simulink model "Controller_implementation"  (R2024a)
settings: Solver=FixedStepAuto  StartTime=0.0  StopTime=inf  RelTol=1e-3  EnableMultiTasking=on
values from neighbouring files (symbols this model uses):
  dis = 81.17 * 10^-3    (= 0.08117)    [Motormixing.m]
  drag_co = torque_Nm / no_rot^2    (= 9.75332775919e-12)    [QuadcopterAttributes.m]
  F = [1 0 0 0 0 0 0 0 ... (first row only)    [LQI_reduced.m]
  g = 9.81    [StateSpace.m]
  K_D_LQR_reduced = lqrd(A_r, B_r, Q_reduced, R_reduced, Ts)    [discrete_control.m]
  K_mm = inv(K_mm_FtoU)    [Motormixing.m]
  Ki_D_lqi_reduced_a = K_lqi_reduced_a(:,9:12)    [discrete_control.m]
  KV_rating = 2800    [QuadcopterAttributes.m]
  Kx_D_lqi_reduced_a = K_lqi_reduced_a(:,1:8)    [discrete_control.m]
  lift_co = thrust_N / no_rot^2    (= 5.88883004597e-10)    [QuadcopterAttributes.m]
  m = 0.5    [StateSpace.m]
  R_kalman = diag([variance_Height, variance_rollAngle, variance_pitchAngle, variance_Yaw, variance_GyroRoll, variance_GyroPitch, variance_GyroYaw])    [BBB_calibration_dev2.m]    (also in Kalman.m = [1 0 0 0 0 0 0)
  Ts = 0.01    [discrete_control.m]
undefined symbols (not defined in the file or in its folder): A_r_d, B_r_d, battery_voltage, C_r_d, D_r_d, DiscIntNeverNeededParam, Discrete, Time
libraries: bbblueActuatorLib x4, simulink_extras x2, bbblueSensorLib x2, ctrlSharedLib x1, dspstat3 x1, dspsigops x1
settings Model: SimulationMode=external  ExtModeTrigDuration=100  Creator=Dario  LastModifiedBy=Henrik
settings SolverCC: PositivePriorityOrder=on
settings OptimizationCC: EnhancedBackFolding=on  PassReuseOutputArgsAs=Individual arguments  ZeroExternalMemoryAtStartup=off  ZeroInternalMemoryAtStartup=off  MaxStackSize=64  OptimizeBlockOrder=speed  DifferentSizesBufferReuse=on  OptimizationCustomize=off  EfficientTunableParamExpr=on
settings DebuggingCC: ParameterTunabilityLossMsg=error
settings HardwareCC: ProdBitPerPointer=32  ProdBitPerSizeT=32  ProdBitPerPtrDiffT=32  ProdLargestAtomicInteger=Long  ProdLargestAtomicFloat=Double  ProdWordSize=32  ProdHWDeviceType=ARM Compatible->ARM Cortex
settings SFSimCC: MATLABDynamicMemAlloc=off
settings RTWCC: Description=Embedded Coder  SystemTargetFile=ert.tlc  HardwareBoard=BeagleBone Blue  TLCOptions="-aInlineSetEventsForThisBaseRateFcn=TLC_FALSE -aSuppressMultiTaskScheduler=TLC_FALSE  -aRateBasedStepFcn=0"  TemplateMakefile=ert_default_tmf  Toolchain=GNU GCC BeagleBone Blue
settings CodeAppCC: ForceParamTrailComments=on  IgnoreCustomStorageClasses=off  OperatorAnnotations=on  SimulinkDataObjDesc=on  SFDataObjDesc=on  InsertBlockDesc=on
settings ERTTargetCC: SupportVariableSizeSignals=on  ExtMode=on  ExtModeMexArgs='192.168.7.2' 0 17725

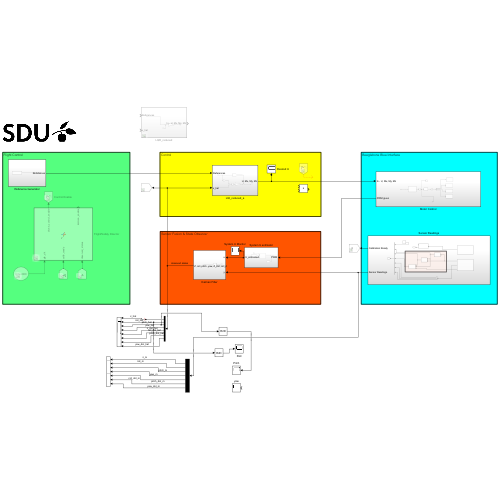
[thumbnail: Simulink's stored preview of the top-level diagram]
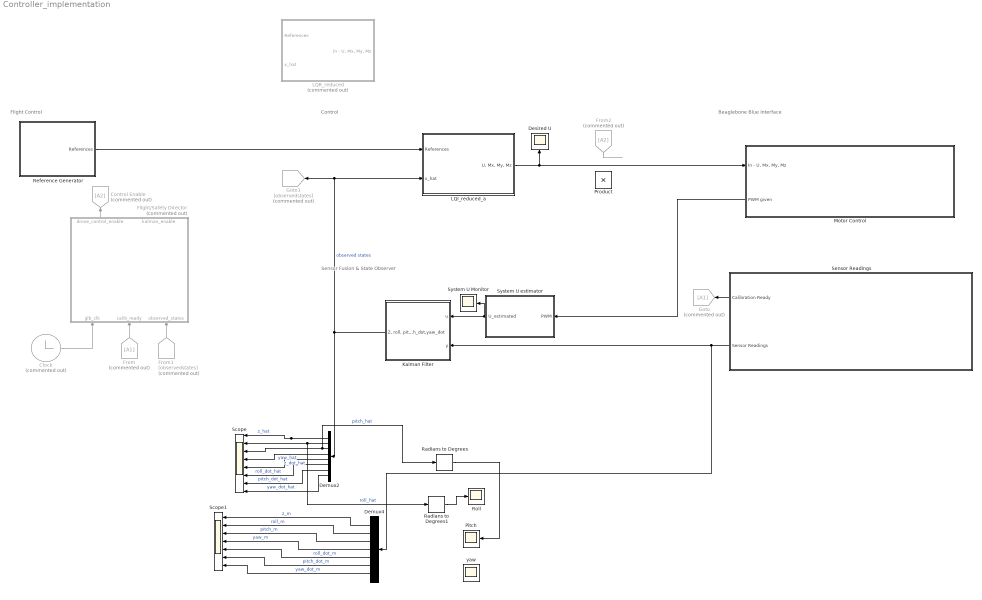
== system Controller_implementation ==
  note: Flight Control
  note: Sensor Fusion & State Observer
  note: Control
  note: Beaglebone Blue Interface
  Clock : Clock  Commented=on
  Control Enable : Goto  Commented=on  GotoTag=A2
  Demux2 : Demux  Outputs=8
  Demux4 : Demux  Outputs=7
  Desired U : Scope
  Flight/Safety Director : MATLAB Function  Commented=on  TreatAsAtomicUnit=on
  From : From  Commented=on  GotoTag=A1
  From1 : From  Commented=on  GotoTag=observedstates
  From2 : From  Commented=on  GotoTag=A2
  Goto : Goto  Commented=on  GotoTag=A1
  Goto1 : Goto  Commented=on  GotoTag=observedstates
  Kalman Filter : Subsystem
  LQI_reduced_a : Subsystem
  LQR_reduced : Subsystem  Commented=on
  Motor Control : Subsystem
      settings: PortSchema="{\"entries\":[{\"content\":{\"sides\":[{\"content\":{\"connectorIds\":[\"In1\",\"Out1\"]},\"type\":\"ConnectorPlacement.EquallySpacedRectSide\",\"uuid\":\"9438d2e9-c32b-4318-b34d-015e09a6ab33\"},{\"content\":{\"side\":\"RIGHT\"},\"type\":\"ConnectorPlacement.EquallySpacedRectSide\",\"uuid\":\"1f1fa985-23a0-47e9-b845-1a4f67fdad51\"},{\"content\":{\"side\":\"TOP\"},\"type\":\"ConnectorPlacement.EquallySpacedRectSide\",\"uuid\":\"e1dcaf73-051b-42d6-8874-ac3417e8774f\"}]},\"type\":\"ConnectorPlacement.EquallySpacedConnector\",\"uuid\":\"43fb11dd-8e84-4752-aa9e-fc065f28cb2c\"}],\"packageUris\":[\"http://schema.mathworks.com/mf0/Connector/R2020b\"],\"version\":\"1.0\"}"
  Pitch : Scope
  Product : Product
  Radians to Degrees : simulink_extras/Transformations/Radians to Degrees
  Radians to Degrees1 : simulink_extras/Transformations/Radians to Degrees
  Reference Generator : Subsystem
  Roll : Scope
  Scope : Scope  NumInputPorts=8
  Scope1 : Scope  NumInputPorts=7
  Sensor Readings : Subsystem
  System U Monitor : Scope
  System U estimator : Subsystem
  yaw : Scope
  wires:
  Reference Generator/1(References) -> LQI_reduced_a/1(References)
  Demux2/1 -> Scope/1  "z_hat"
  Demux2/2 -> Radians to Degrees1/1, Scope/2  "roll_hat"
  Demux2/3 -> Radians to Degrees/1, Scope/3  "pitch_hat"
  Demux2/4 -> Scope/4  "yaw_hat"
  Demux2/5 -> Scope/5  "z_dot_hat"
  Demux2/6 -> Scope/6  "roll_dot_hat"
  Demux2/7 -> Scope/7  "pitch_dot_hat"
  Demux2/8 -> Scope/8  "yaw_dot_hat"
  System U estimator/1(U_estimated) -> Kalman Filter/1(u), System U Monitor/1
  Demux4/3 -> Scope1/3  "pitch_m"
  Demux4/5 -> Scope1/5  "roll_dot_m"
  Demux4/7 -> Scope1/7  "yaw_dot_m"
  Demux4/6 -> Scope1/6  "pitch_dot_m"
  Demux4/2 -> Scope1/2  "roll_m"
  Demux4/1 -> Scope1/1  "z_m"
  Demux4/4 -> Scope1/4  "yaw_m"
  Radians to Degrees/1 -> Pitch/1
  Radians to Degrees1/1 -> Roll/1
  Sensor Readings/2(Sensor Readings) -> Demux4/1, Kalman Filter/2(y)
  Motor Control/1(PWM given) -> System U estimator/1(PWM)
  Kalman Filter/1("Z, roll, pitch, yaw, Z_dot, roll_dot, pitch_dot,yaw_dot") -> Demux2/1, LQI_reduced_a/2(x_hat), Goto1/1  "observed states"
  Sensor Readings/1(Calibration Ready) -> Goto/1
  From/1 -> Flight/Safety Director/2(calib_ready)
  From1/1 -> Flight/Safety Director/3(observed_states)
  LQI_reduced_a/1("U, Mx, My, Mz") -> Desired U/1, Motor Control/1("In - U, Mx, My, Mz")
  Flight/Safety Director/1(drone_control_enable) -> Control Enable/1
  From2/1 -> ?
  Clock/1 -> Flight/Safety Director/1(glb_clk)

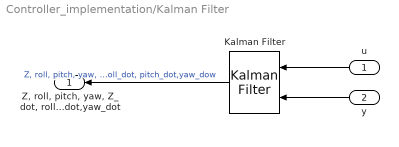
== system Controller_implementation/Kalman Filter ==
  u : Inport
  y : Inport  Port=2
  Kalman Filter : ctrlSharedLib/Kalman Filter  TimeDomain=Discrete-Time  UseCurrentEstimator=on  ModelSource=Individual A, B, C, D matrices  ModelSourceVariable=ss(0.95,1,1,0,1)  A=A_r_d  B=B_r_d  C=C_r_d  D=D_r_d  NumberOfStates=1  NumberOfInputs=1  NumberOfOutputs=1  InitialEstimateSource=Dialog  X0=0  P0=10  UseK=off  UseGH=off  NumberOfProcessNoiseInputs=1  G=1  TimeInvariantG=on  H=0  TimeInvariantH=on  Q=Q_kalman_d  TimeInvariantQ=on  R=R_kalman  TimeInvariantR=on  N=0  TimeInvariantN=on  AddInputPort=on  AddEnablePort=off  OutputEstimatedY=off  OutputP=off  Ts=Ts
  "Z, roll, pitch, yaw, Z_dot, roll_dot, pitch_dot,yaw_dot" : Outport
  wires:
  y/1 -> Kalman Filter/2
  u/1 -> Kalman Filter/1
  Kalman Filter/1 -> "Z, roll, pitch, yaw, Z_dot, roll_dot, pitch_dot,yaw_dot"/1  "Z, roll, pitch, yaw, Z_dot, roll_dot, pitch_dot,yaw_dow"

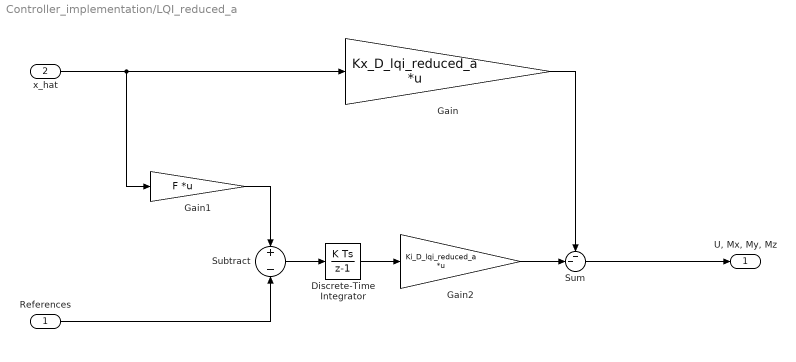
== system Controller_implementation/LQI_reduced_a ==
  References : Inport
  x_hat : Inport  Port=2
  Discrete-Time Integrator : DiscreteIntegrator  SampleTime=Ts  ICPrevOutput=DiscIntNeverNeededParam  ICPrevScaledInput=DiscIntNeverNeededParam
  Gain : Gain  Gain=Kx_D_lqi_reduced_a  Multiplication=Matrix(K*u)
  Gain1 : Gain  Gain=F  Multiplication=Matrix(K*u)
  Gain2 : Gain  Gain=Ki_D_lqi_reduced_a  Multiplication=Matrix(K*u)
  Subtract : Sum  Inputs=+-
  Sum : Sum  Inputs=--|
  "U, Mx, My, Mz" : Outport
  wires:
  Subtract/1 -> Discrete-Time Integrator/1
  Gain1/1 -> Subtract/1
  Sum/1 -> "U, Mx, My, Mz"/1
  Gain/1 -> Sum/1
  Gain2/1 -> Sum/2
  Discrete-Time Integrator/1 -> Gain2/1
  References/1 -> Subtract/2
  x_hat/1 -> Gain/1, Gain1/1

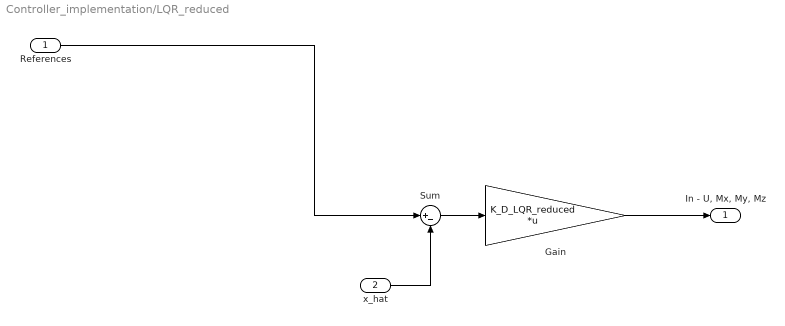
== system Controller_implementation/LQR_reduced ==
  References : Inport
  x_hat : Inport  Port=2
  Gain : Gain  Gain=K_D_LQR_reduced  Multiplication=Matrix(K*u)
  Sum : Sum  Inputs=|+-
  "In - U, Mx, My, Mz" : Outport
  wires:
  Gain/1 -> "In - U, Mx, My, Mz"/1
  Sum/1 -> Gain/1
  References/1 -> Sum/1
  x_hat/1 -> Sum/2

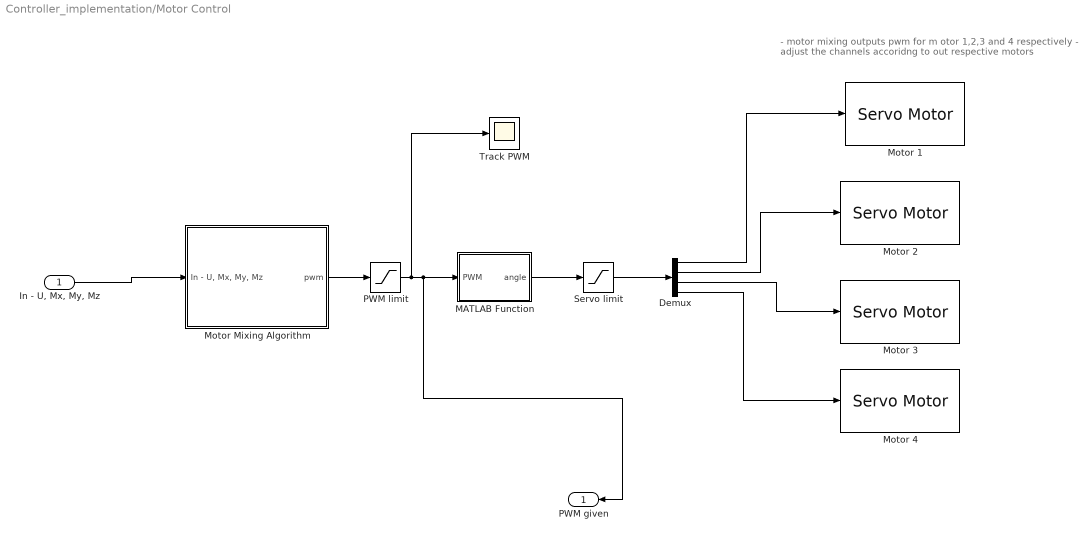
== system Controller_implementation/Motor Control ==
  note: - motor mixing outputs pwm for m otor 1,2,3 and 4 respectively
      | - adjust the channels accoridng to out respective motors
  "In - U, Mx, My, Mz" : Inport
  Demux : Demux
  MATLAB Function : MATLAB Function  TreatAsAtomicUnit=on
  Motor 1 : bbblueActuatorLib/Servo Motor  channel=1  SimulateUsing=Code generation
  Motor 2 : bbblueActuatorLib/Servo Motor  channel=2  SimulateUsing=Code generation
  Motor 3 : bbblueActuatorLib/Servo Motor  channel=3  SimulateUsing=Code generation
  Motor 4 : bbblueActuatorLib/Servo Motor  channel=4  SimulateUsing=Code generation
  Motor Mixing Algorithm : Subsystem
  PWM limit : Saturate  UpperLimit=255  LowerLimit=0
  Servo limit : Saturate  UpperLimit=180  LowerLimit=0
  Track PWM : Scope
  PWM given : Outport
  wires:
  Servo limit/1 -> Demux/1
  PWM limit/1 -> Track PWM/1, PWM given/1, MATLAB Function/1(PWM)
  Demux/4 -> Motor 4/1
  Demux/1 -> Motor 1/1
  Demux/2 -> Motor 2/1
  Motor Mixing Algorithm/1(pwm) -> PWM limit/1
  Demux/3 -> Motor 3/1
  MATLAB Function/1(angle) -> Servo limit/1
  "In - U, Mx, My, Mz"/1 -> Motor Mixing Algorithm/1("In - U, Mx, My, Mz")

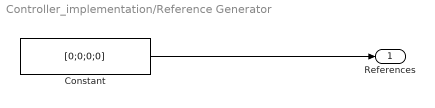
== system Controller_implementation/Reference Generator ==
  Constant : Constant  Value=[0;0;0;0]
  References : Outport
  wires:
  Constant/1 -> References/1

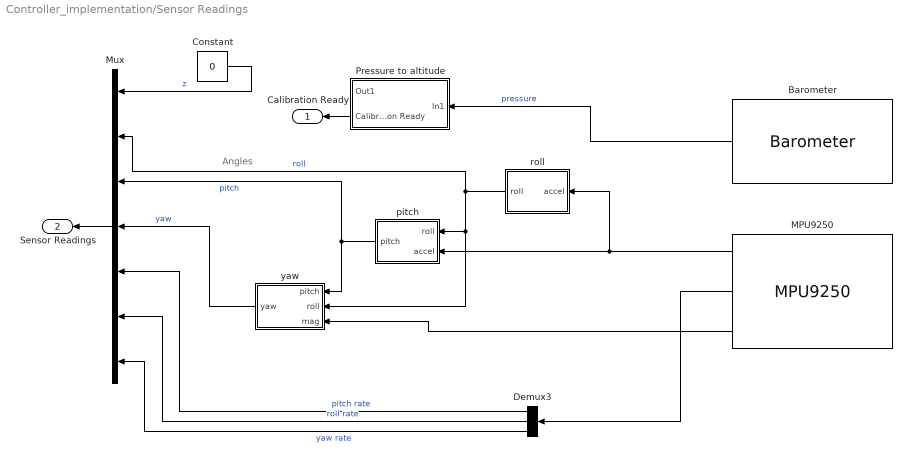
== system Controller_implementation/Sensor Readings ==
  note: Angles
  Barometer : bbblueSensorLib/Barometer  OSRSelection=1  IIRFilterCoeff=Off  SampleTime=Ts
  Constant : Constant  Value=0
  Demux3 : Demux  Outputs=3
  MPU9250 : bbblueSensorLib/MPU9250  OperationMode=DMP  Accel=on  AngularRate=on  Ak8963Field=on  EulerAngles=off  Quat=off  AccelRange=2G  Acceldlpf=1  GyroRange=250 dps  Gyrodlpf=1  DmpOdr=200 Hz  SampleTime=Ts
  Mux : Mux  Inputs=7
  Pressure to altitude : Subsystem
  pitch : MATLAB Function  TreatAsAtomicUnit=on
  "roll " : MATLAB Function  TreatAsAtomicUnit=on
  yaw : MATLAB Function  TreatAsAtomicUnit=on
  Calibration Ready : Outport
  Sensor Readings : Outport  Port=2
  wires:
  Demux3/3 -> Mux/7  "yaw rate"
  yaw/1(yaw) -> Mux/4  "yaw"
  Constant/1 -> Mux/1  "z"
  MPU9250/3 -> yaw/3(mag)
  MPU9250/2 -> Demux3/1
  Demux3/2 -> Mux/6  "roll rate"
  Demux3/1 -> Mux/5  "pitch rate"
  "roll "/1(roll) -> yaw/2(roll), pitch/1(roll), Mux/2  "roll"
  Barometer/1 -> Pressure to altitude/1(In1)  "pressure"
  pitch/1(pitch) -> yaw/1(pitch), Mux/3  "pitch"
  Mux/1 -> Sensor Readings/1
  Pressure to altitude/2(Calibration Ready) -> Calibration Ready/1
  MPU9250/1 -> "roll "/1(accel), pitch/2(accel)

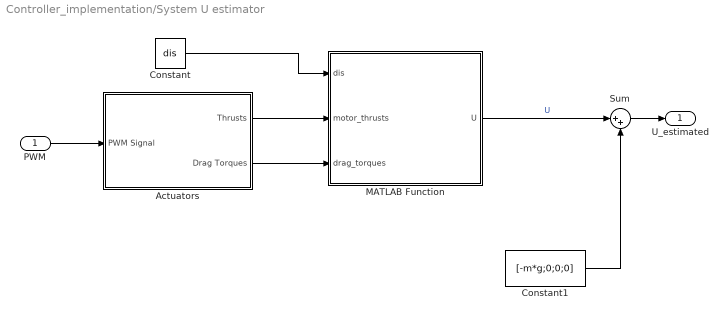
== system Controller_implementation/System U estimator ==
  PWM : Inport
  Actuators : Subsystem
  Constant : Constant  Value=dis
  Constant1 : Constant  Value=[-m*g;0;0;0]  SampleTime=Ts
  MATLAB Function : MATLAB Function  TreatAsAtomicUnit=on
  Sum : Sum  Inputs=|++
  U_estimated : Outport
  wires:
  PWM/1 -> Actuators/1(PWM Signal)
  Actuators/1(Thrusts) -> MATLAB Function/2(motor_thrusts)
  Constant/1 -> MATLAB Function/1(dis)
  Actuators/2(Drag Torques) -> MATLAB Function/3(drag_torques)
  MATLAB Function/1(U) -> Sum/1  "U"
  Constant1/1 -> Sum/2
  Sum/1 -> U_estimated/1

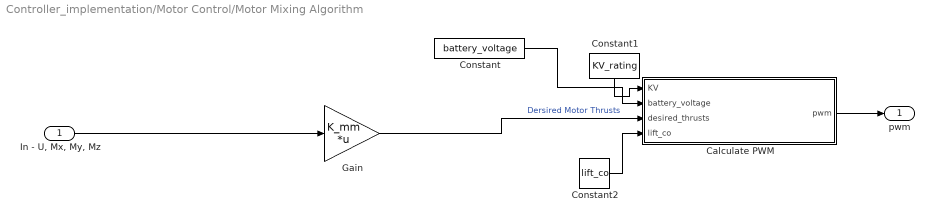
== system Controller_implementation/Motor Control/Motor Mixing Algorithm ==
  "In - U, Mx, My, Mz" : Inport
  Calculate PWM : MATLAB Function  TreatAsAtomicUnit=on
  Constant : Constant  Value=battery_voltage
  Constant1 : Constant  Value=KV_rating
  Constant2 : Constant  Value=lift_co
  Gain : Gain  Gain=K_mm  Multiplication=Matrix(K*u)
  pwm : Outport
  wires:
  "In - U, Mx, My, Mz"/1 -> Gain/1
  Gain/1 -> Calculate PWM/3(desired_thrusts)  "Dersired Motor Thrusts"
  Constant/1 -> Calculate PWM/2(battery_voltage)
  Constant1/1 -> Calculate PWM/1(KV)
  Calculate PWM/1(pwm) -> pwm/1
  Constant2/1 -> Calculate PWM/4(lift_co)

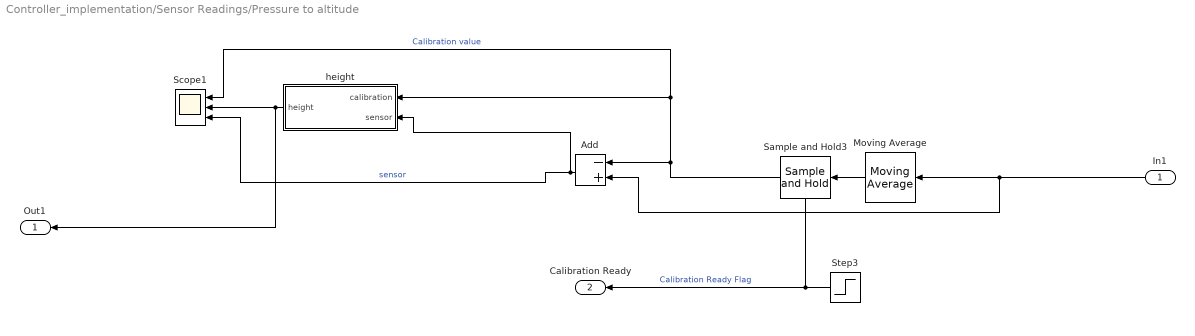
== system Controller_implementation/Sensor Readings/Pressure to altitude ==
  In1 : Inport
  Add : Sum  Inputs=-+
  Moving Average : dspstat3/Moving Average  Method=Exponential weighting  ForgettingFactorPort=off  SpecifyWindowLength=on  WindowLength=4  OverlapLength=3  AllowArbitraryInputLength=off  ForgettingFactor=1.0  SimulateUsing=Code generation
  Sample and Hold3 : dspsigops/Sample and Hold  trig=Rising edge  initCond=100000000  latchinput=off
  Scope1 : Scope  NumInputPorts=3
  Step3 : Step  Time=5  SampleTime=Ts
  height : MATLAB Function  TreatAsAtomicUnit=on
  Out1 : Outport
  Calibration Ready : Outport  Port=2
  wires:
  height/1(height) -> Out1/1, Scope1/2
  Moving Average/1 -> Sample and Hold3/1
  Sample and Hold3/1 -> Scope1/1, height/1(calibration), Add/1  "Calibration value"
  In1/1 -> Add/2, Moving Average/1
  Step3/1 -> Calibration Ready/1, Sample and Hold3/Trigger  "Calibration Ready Flag"
  Add/1 -> height/2(sensor), Scope1/3  "sensor"

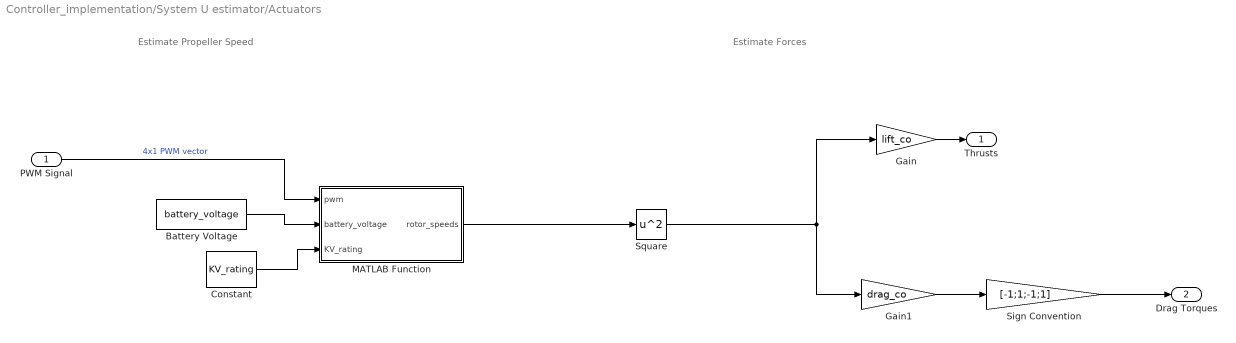
== system Controller_implementation/System U estimator/Actuators ==
  note: Estimate Forces
  note: Estimate Propeller Speed
  PWM Signal : Inport
  Battery Voltage : Constant  Value=battery_voltage  SampleTime=Ts
  Constant : Constant  Value=KV_rating  SampleTime=Ts
  Gain : Gain  Gain=lift_co
  Gain1 : Gain  Gain=drag_co
  MATLAB Function : MATLAB Function  TreatAsAtomicUnit=on
  Sign Convention : Gain  Gain=[-1;1;-1;1]
  Square : Math  Operator=square
  Thrusts : Outport
  Drag Torques : Outport  Port=2
  wires:
  Constant/1 -> MATLAB Function/3(KV_rating)
  Battery Voltage/1 -> MATLAB Function/2(battery_voltage)
  PWM Signal/1 -> MATLAB Function/1(pwm)  "4x1 PWM vector"
  MATLAB Function/1(rotor_speeds) -> Square/1
  Gain/1 -> Thrusts/1
  Square/1 -> Gain/1, Gain1/1
  Gain1/1 -> Sign Convention/1
  Sign Convention/1 -> Drag Torques/1

== matlab function Controller_implementation/System U estimator/Actuators/MATLAB Function ==
  data: pwm input; rotor_speeds output; battery_voltage input; KV_rating input
function rotor_speeds = fcn(pwm, battery_voltage, KV_rating)
    
    rotor_speeds = zeros(4,1); % Initialize rotor_speeds
    
    for i = 1:1:4
    
        duty_cycle = pwm(i,1)/255;
        rotor_speeds(i,1) = duty_cycle * battery_voltage * KV_rating;
    
    end

end

== matlab function Controller_implementation/Motor Control/MATLAB Function ==
  data: PWM input; angle output
function angle = fcn(PWM)

angle = (180/255)*PWM;

== matlab function Controller_implementation/Motor Control/Motor Mixing Algorithm/Calculate PWM ==
  data: KV input; battery_voltage input; desired_thrusts input; pwm output; lift_co input
function pwm = calc_PWM(KV, battery_voltage, desired_thrusts, lift_co)

    pwm = zeros(4,1);
    req_rotorspeed = zeros (4,1);
    max_possible_rot_speed = battery_voltage * KV;

    for i = 1:1:4
        if desired_thrusts(i,1) > 0
            req_rotorspeed(i,1) = sqrt(desired_thrusts(i,1)/lift_co); % Estimate required rotor speeds
        else
            req_rotorspeed(i,1) = 0;
        end
        dutycycle = req_rotorspeed(i,1) / max_possible_rot_speed;
        pwm(i,1) = dutycycle * 255;
        
    end

== matlab function Controller_implementation/Sensor Readings/roll  ==
  data: roll output; accel input
function roll = roll(accel)

Ay = accel(2);
Az = accel(3);

%roll = atan(sqrt(Ax^2 + Ay^2)/Az);
%if first one doesn work, use this
roll = atan(Ay/Az);

== matlab function Controller_implementation/Sensor Readings/pitch ==
  data: roll input; pitch output; accel input
function pitch = pitch(roll, accel)

Ax = accel(1);
Ay = accel(2);
Az = accel(3);

Gz2 = Ay * sin(roll) + Az * cos(roll);

%pitch = 
%pitch = atan(Ax/sqrt(Ay^2 + Az^2));
%if first one doesnt work use this
pitch = atan(-Ax/Gz2);

== matlab function Controller_implementation/Sensor Readings/yaw ==
  data: pitch input; roll input; mag input; yaw output
function yaw = yaw(pitch, roll, mag)

    Bx = mag(1);
    By = mag(2);
    Bz = mag(3);

    By2 = Bz * sin(roll) - By * cos(roll);
    Bz2 = By * sin(roll) + Bz * cos(roll);
    Bx3 = Bx * cos(pitch) + Bz2 * sin(pitch);

    yaw = atan2(By2,Bx3);
%{
x = mag(1);
y = mag(2);

yaw = atan(x/y);

%}

== matlab function Controller_implementation/Sensor Readings/Pressure to altitude/height ==
  data: calibration input; sensor input; height output
function height = fcn(calibration,sensor)

% barometic formula

height = -(sensor/calibration)*8430 ;

== matlab function Controller_implementation/System U estimator/MATLAB Function ==
  data: dis input; motor_thrusts input; U output; drag_torques input
function U = calc_U(dis, motor_thrusts, drag_torques)

    U = zeros(4,1); % Init U

    U(1,1) = sum(motor_thrusts); % Overall Thrust
    U(2,1) = dis * (motor_thrusts(1,1) + motor_thrusts(2,1) - (motor_thrusts(3,1) + motor_thrusts(4,1))); % Mx
    U(3,1) = dis * (motor_thrusts(2,1) + motor_thrusts(3,1) - (motor_thrusts(1,1) + motor_thrusts(4,1))); % My
    U(4,1) = sum(drag_torques); % Mz

== matlab function Controller_implementation/Flight//Safety Director ==
  data: glb_clk input; calib_ready input; drone_control_enable output; observed_states input; kalman_enable output
function [drone_control_enable, kalman_enable]= fcn(glb_clk, calib_ready, observed_states)

% drone_control_enable = 1; % Enable controller

% Read in states
z_hat = observed_states(1);
roll_hat = observed_states(2) * 180/pi; 
pitch_hat = observed_states(3) * 180/pi;
yaw_hat = observed_states(4) * 180/pi;
z_dot_hat = observed_states(5);
roll_dot_hat = observed_states(6);
pitch_dot_hat = observed_states(7);
yaw_dot_hat = observed_states(8);


% Constraints
max_ang = 30;
min_ang = -max_ang;

if (roll_hat > max_ang) || (pitch_hat > max_ang) || (roll_hat < min_ang) || (pitch_hat < min_ang)

    drone_control_enable = 0; % Cut of controller

elseif calib_ready

    drone_control_enable = 1;
    kalman_enable = 1;

end
